simulink model "pendulum_sol"  (R2023b)
settings: Solver=ode3  StartTime=0.0  StopTime=10.0  FixedStep=0.01  RelTol=1e-3
values from neighbouring files (symbols this model uses):
  A = [ 0 1 ; -g/l*cos(pi/4) -d/(m*l^2) ]    [pendulum_par_sol.m]
  a = [ m ; g ; l ; d ]    [pendulum_par_sol.m]
  B = [ 0 ; 1/(m*l^2) ]    [pendulum_par_sol.m]
  ustar = m*g*l*sin(xstar(1))    [pendulum_par_sol.m]
  xstar = [ pi/4 ; 0 ]    [pendulum_par_sol.m]
libraries: simulink_extras x4
settings Model: Creator=jerome  LastModifiedBy=jerome
settings ModelReferenceCC: EnableRefExpFcnMdlSchedulingChecks=on

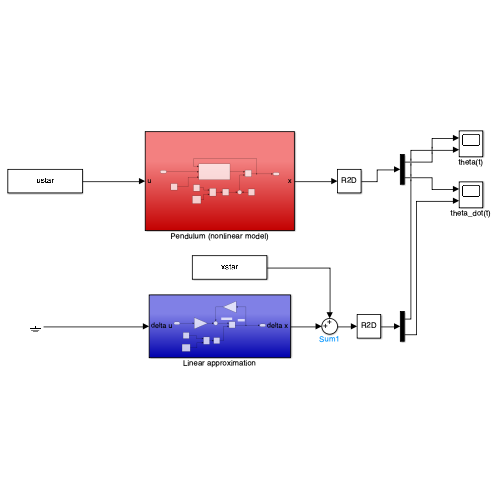
[thumbnail: Simulink's stored preview of the top-level diagram]
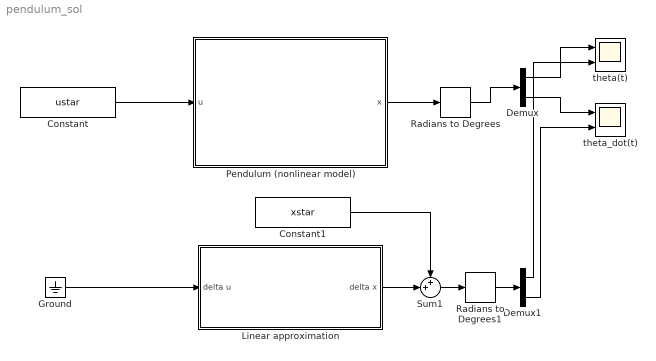
== system pendulum_sol ==
  Constant : Constant  Value=ustar
  Constant1 : Constant  Value=xstar  VectorParams1D=off
  Demux : Demux  Outputs=2
  Demux1 : Demux  Outputs=2
  Ground : Ground
  Linear approximation : Subsystem
  Pendulum (nonlinear model) : Subsystem
  Radians to Degrees : simulink_extras/Transformations/Radians to Degrees
  Radians to Degrees1 : simulink_extras/Transformations/Radians to Degrees
  Sum1 : Sum  Inputs=++|
  theta(t) : Scope  NumInputPorts=2
  theta_dot(t) : Scope  NumInputPorts=2
  wires:
  Constant/1 -> Pendulum (nonlinear model)/1(u)
  Pendulum (nonlinear model)/1(x) -> Radians to Degrees/1
  Radians to Degrees/1 -> Demux/1
  Demux/1 -> theta(t)/1
  Demux/2 -> theta_dot(t)/1
  Constant1/1 -> Sum1/1
  Sum1/1 -> Radians to Degrees1/1
  Demux1/1 -> theta(t)/2
  Radians to Degrees1/1 -> Demux1/1
  Demux1/2 -> theta_dot(t)/2
  Ground/1 -> Linear approximation/1(delta u)
  Linear approximation/1(delta x) -> Sum1/2

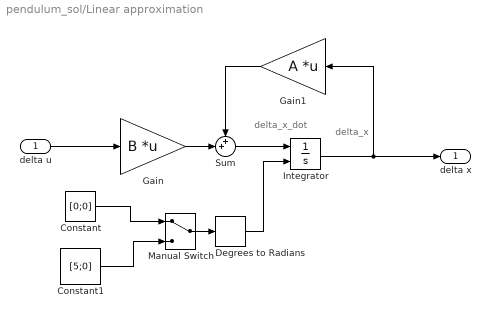
== system pendulum_sol/Linear approximation ==
  note: delta_x_dot
  note: delta_x
  delta u : Inport
  Constant : Constant  Value=[0;0]  VectorParams1D=off
  Constant1 : Constant  Value=[5;0]  VectorParams1D=off
  Degrees to Radians : simulink_extras/Transformations/Degrees to Radians
  Gain : Gain  Gain=B  Multiplication=Matrix(K*u) (u vector)
  Gain1 : Gain  Gain=A  Multiplication=Matrix(K*u) (u vector)
  Integrator : Integrator  InitialConditionSource=external  InitialCondition=[0.5;0]
  Manual Switch : ManualSwitch
  Sum : Sum  Inputs=++|
  delta x : Outport
  wires:
  delta u/1 -> Gain/1
  Sum/1 -> Integrator/1
  Integrator/1 -> Gain1/1, delta x/1
  Gain1/1 -> Sum/1
  Gain/1 -> Sum/2
  Manual Switch/1 -> Degrees to Radians/1
  Constant/1 -> Manual Switch/1
  Constant1/1 -> Manual Switch/2
  Degrees to Radians/1 -> Integrator/2

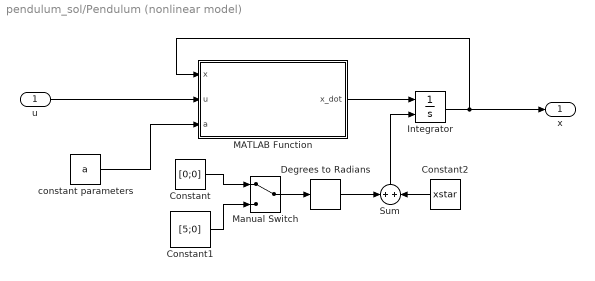
== system pendulum_sol/Pendulum (nonlinear model) ==
  u : Inport
  Constant : Constant  Value=[0;0]  VectorParams1D=off
  Constant1 : Constant  Value=[5;0]  VectorParams1D=off
  Constant2 : Constant  Value=xstar  VectorParams1D=off
  Degrees to Radians : simulink_extras/Transformations/Degrees to Radians
  Integrator : Integrator  InitialConditionSource=external  InitialCondition=xstar
  MATLAB Function : MATLAB Function  TreatAsAtomicUnit=on
  Manual Switch : ManualSwitch
  Sum : Sum
  constant parameters : Constant  Value=a  VectorParams1D=off
  x : Outport
  wires:
  u/1 -> MATLAB Function/2(u)
  MATLAB Function/1(x_dot) -> Integrator/1
  Integrator/1 -> MATLAB Function/1(x), x/1
  constant parameters/1 -> MATLAB Function/3(a)
  Constant/1 -> Manual Switch/1
  Constant1/1 -> Manual Switch/2
  Manual Switch/1 -> Degrees to Radians/1
  Sum/1 -> Integrator/2
  Constant2/1 -> Sum/2
  Degrees to Radians/1 -> Sum/1

== matlab function pendulum_sol/Pendulum (nonlinear model)/MATLAB Function ==
  data: x input; u input; x_dot output; a input
function x_dot = f(x,u,a)

% a is the vector of constant parameters
m = a(1);
g = a(2);
l = a(3);
d = a(4);

x_dot = [ x(2) ; 1/(m*l^2)*(-m*g*l*sin(x(1))-d*x(2)+u) ];
